simulink model "virtual_oscilloscope"  (R2020a)
settings: Solver=FixedStepAuto  StartTime=0.0  StopTime=inf  FixedStep=1  RelTol=1e-3  EnableMultiTasking=on
InitFcn:
  | update_comport
undefined symbols (not defined in the file or in its folder): serial
libraries: instrumentlib x3, simulink x1, dspspect3 x1
settings Model: Creator=domanico  LastModifiedBy=plyoung
settings DataIOCC: LimitDataPoints=on  ReturnWorkspaceOutputs=off
settings OptimizationCC: LifeSpan=inf
settings DebuggingCC: AllowSymbolicDim=off  SFUnexpectedBacktrackingDiag=warning  SFNoUnconditionalDefaultTransitionDiag=warning  SFExecutionAtInitializationDiag=none  ArithmeticOperatorsInVariantConditions=warning
settings ModelReferenceCC: PropagateSignalLabelsOutOfModel=off
settings SFSimCC: SimUseLocalCustomCode=off  CustomCodeUndefinedFunction=UseInterfaceOnly
settings RTWCC: RTWUseLocalCustomCode=off
settings CodeAppCC: StateflowObjectComments=on
settings GRTTargetCC: TargetLangStandard=C89/C90 (ANSI)
settings ConfigComp: CovMetricSettings=dw  CovHtmlReporting=on  CovSaveCumulativeToWorkspaceVar=on  CovSaveSingleToWorkspaceVar=on  CovExternalEMLEnable=off

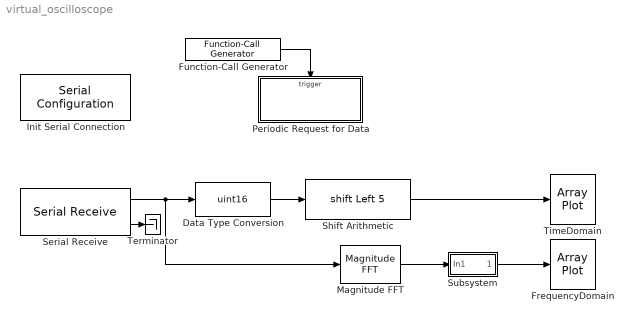
== system virtual_oscilloscope ==
  Data Type Conversion : DataTypeConversion  OutDataTypeStr=uint16
  FrequencyDomain : ArrayPlot
  Function-Call Generator : simulink/Ports & Subsystems/Function-Call Generator  sample_time=1  numberOfIterations=1
  Init Serial Connection : instrumentlib/Serial Configuration  Priority=-200000  ComPortMenu=COM2  ComPort=COM4  ObjConstructor=serial('COM4');  BaudRate=9600  DataBits=8  Parity=none  StopBits=1  FlowControl=none  Timeout=10  ByteOrder=LittleEndian
  Magnitude FFT : dspspect3/Magnitude FFT  mag_or_magsq=Magnitude squared  FFTImplementation=Auto  fftLenInherit=on  fftsize=256  WrapInput=on
      settings: SourceProductBaseCode=DS
  Periodic Request for Data : Subsystem  TreatAsAtomicUnit=on
  Serial Receive : instrumentlib/Serial Receive  ComPortMenu=COM2  ComPort=COM4  ObjConstructor=serial('COM4');  Terminator=<none>  DataSize=512  DataType=uint8  EnableBlockingMode=off  ActionDataUnavailable=Output last received value  CustomValue=0  SampleTime=1
  Shift Arithmetic : ArithShift  BitShiftNumber=5  BitShiftDirection=Left
  Subsystem : Subsystem
  Terminator : Terminator
  TimeDomain : ArrayPlot
  wires:
  Function-Call Generator/1 -> Periodic Request for Data/Trigger
  Shift Arithmetic/1 -> TimeDomain/1
  Serial Receive/2 -> Terminator/1
  Serial Receive/1 -> Magnitude FFT/1, Data Type Conversion/1
  Data Type Conversion/1 -> Shift Arithmetic/1
  Magnitude FFT/1 -> Subsystem/1(In1)
  Subsystem/1(Out1) -> FrequencyDomain/1

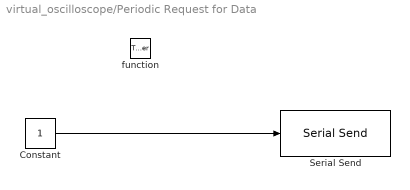
== system virtual_oscilloscope/Periodic Request for Data ==
  function : TriggerPort  TriggerType=function-call  VariantControl=(inherit)
  Constant : Constant
  Serial Send : instrumentlib/Serial Send  ComPortMenu=COM2  ComPort=COM4  ObjConstructor=serial('COM4');  Terminator=<none>  EnableBlockingMode=on
  wires:
  Constant/1 -> Serial Send/1

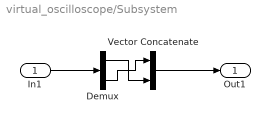
== system virtual_oscilloscope/Subsystem ==
  In1 : Inport
  Demux : Demux  Outputs=2
  Vector Concatenate : Concatenate
  Out1 : Outport
  wires:
  In1/1 -> Demux/1
  Demux/2 -> Vector Concatenate/1
  Vector Concatenate/1 -> Out1/1
  Demux/1 -> Vector Concatenate/2
